simulink model "velocity"  (R2018b)
settings: Solver=VariableStepAuto  StartTime=0.0  StopTime=10.0  RelTol=1e-3
settings Model: Creator=Dominik  LastModifiedBy=Dominik

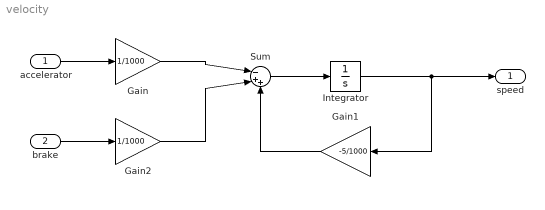
== system velocity ==
  "accelerator " : Inport
  brake : Inport  Port=2
  Gain : Gain  Gain=1/1000
  Gain1 : Gain  Gain=-5/1000
  Gain2 : Gain  Gain=1/1000
  Integrator : Integrator
  Sum : Sum  Inputs=|-++
  "speed " : Outport
  wires:
  "accelerator "/1 -> Gain/1
  Sum/1 -> Integrator/1
  Integrator/1 -> Gain1/1, "speed "/1
  Gain1/1 -> Sum/3
  brake/1 -> Gain2/1
  Gain2/1 -> Sum/2
  Gain/1 -> Sum/1
